simulink model "Control_Adap_1"  (R2021b)
settings: Solver=VariableStepAuto  StartTime=0.0  StopTime=50  RelTol=1e-3
settings Model: Creator=Alejandro  LastModifiedBy=cesar

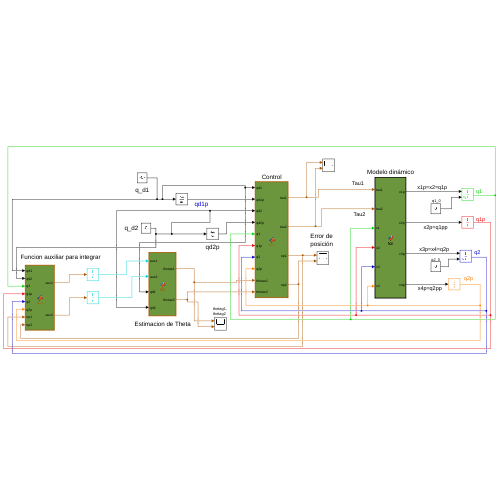
[thumbnail: Simulink's stored preview of the top-level diagram]
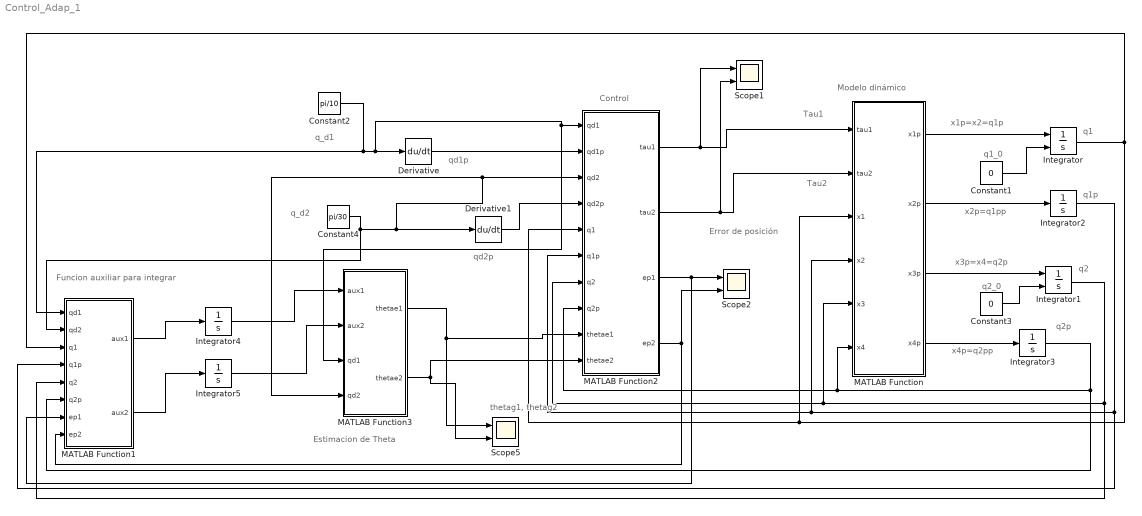
== system Control_Adap_1 ==
  note: Modelo dinámico
  note: q1_0
  note: q2p
  note: q2
  note: q1
  note: q_d2
  note: x3p=x4=q2p
  note: x2p=q1pp
  note: Tau2
  note: Error de posición
  note: x1p=x2=q1p
  note: x4p=q2pp
  note: Control
  note: qd1p
  note: Tau1
  note: q_d1
  note: qd2p
  note: q1p
  note: q2_0
  note: thetag1, thetag2
  note: Estimacion de Theta
  note: Funcion auxiliar para integrar
  Constant1 : Constant  Value=0
  Constant2 : Constant  Value=pi/10
  Constant3 : Constant  Value=0
  Constant4 : Constant  Value=pi/30
  Derivative : Derivative
  Derivative1 : Derivative
  Integrator : Integrator  InitialConditionSource=external
  Integrator1 : Integrator  InitialConditionSource=external
  Integrator{2..5} (4 alike) : Integrator
  MATLAB Function : MATLAB Function  TreatAsAtomicUnit=on
  MATLAB Function1 : MATLAB Function  TreatAsAtomicUnit=on
  MATLAB Function2 : MATLAB Function  TreatAsAtomicUnit=on
  MATLAB Function3 : MATLAB Function  TreatAsAtomicUnit=on
  Scope1 : Scope  NumInputPorts=2
  Scope2 : Scope  NumInputPorts=2
  Scope5 : Scope  NumInputPorts=2
  wires:
  Constant4/1 -> MATLAB Function1/2(qd2), Derivative1/1, MATLAB Function2/3(qd2), MATLAB Function3/4(qd2)
  Derivative/1 -> MATLAB Function2/2(qd1p)
  MATLAB Function3/1(thetae1) -> MATLAB Function2/9(thetae1), Scope5/1
  MATLAB Function2/1(tau1) -> Scope1/1, MATLAB Function/1(tau1)
  Constant2/1 -> MATLAB Function1/1(qd1), Derivative/1, MATLAB Function3/3(qd1), MATLAB Function2/1(qd1)
  MATLAB Function/4(x4p) -> Integrator3/1
  Constant3/1 -> Integrator1/2
  Integrator2/1 -> MATLAB Function1/4(q1p), MATLAB Function/4(x2), MATLAB Function2/6(q1p)
  MATLAB Function2/2(tau2) -> Scope1/2, MATLAB Function/2(tau2)
  Constant1/1 -> Integrator/2
  Integrator/1 -> MATLAB Function1/3(q1), MATLAB Function2/5(q1), MATLAB Function/3(x1)
  MATLAB Function/2(x2p) -> Integrator2/1
  MATLAB Function/3(x3p) -> Integrator1/1
  MATLAB Function/1(x1p) -> Integrator/1
  Integrator3/1 -> MATLAB Function1/6(q2p), MATLAB Function2/8(q2p), MATLAB Function/6(x4)
  Derivative1/1 -> MATLAB Function2/4(qd2p)
  Integrator1/1 -> MATLAB Function1/5(q2), MATLAB Function/5(x3), MATLAB Function2/7(q2)
  Integrator4/1 -> MATLAB Function3/1(aux1)
  MATLAB Function1/1(aux1) -> Integrator4/1
  MATLAB Function1/2(aux2) -> Integrator5/1
  Integrator5/1 -> MATLAB Function3/2(aux2)
  MATLAB Function3/2(thetae2) -> MATLAB Function2/10(thetae2), Scope5/2
  MATLAB Function2/3(ep1) -> MATLAB Function1/7(ep1), Scope2/1
  MATLAB Function2/4(ep2) -> Scope2/2, MATLAB Function1/8(ep2)

== matlab function Control_Adap_1/MATLAB Function1 ==
  data: qd1 input; qd2 input; q1 input; q1p input; q2 input; q2p input; aux1 output; aux2 output; ep1 input; ep2 input
function [aux1,aux2]= fcn(qd1,qd2,q1,q1p,q2,q2p,ep1,ep2)
% Parámetros
m1=6.5225;l1=0.26;lc1=0.0983;
g=9.81;I1=0.1213;
e0=5;
%---ERROR PARA EL ESLABÓN 1 ------
ep1=qd1-q1;     %qtilde
%ev1=qd1p-q1p;   %qtildepunto
%---ERROR PARA EL ESLABÓN 2 ------
ep2=qd2-q2;     %qtilde
%ev2=qd2p-q2p;   %qtildepunto
%------- VECTOR DE  ERROR DE POSICIÓN ------
ep=[ ep1;ep2];
%------- VECTOR DE  QP ------
qp=[ q1p;q2p];  
%---------- MATRIZ PHI_G -----------------------
phig=[l1*g*sin(qd1)   g*sin(qd1+qd2);
            0          g*sin(qd1+qd2)];    
a=l1*g*sin(qd1);
b=g*sin(qd1+qd2);
%------- Calcular de la variable auxiliar --------------
aux1=(e0/(1+norm(ep)))*(ep1-q1p);
aux2=(e0/(1+norm(ep)))*(ep2-q2p);

== matlab function Control_Adap_1/MATLAB Function ==
  data: tau1 input; x1p output; tau2 input; x1 input; x2 input; x3 input; x4 input; x2p output; x3p output; x4p output
function  [x1p,x2p,x3p,x4p] = fcn(tau1,tau2,x1,x2,x3,x4)
% Parámetros
m1=6.5225;I1=0.1213;
I2=0.0116;l1=0.26;
lc1=0.0983;lc2=0.0229;g=9.81;
qd1 = pi/10;
m2=2.0458;
l2 = 0.26;
%-------------------------------------------
M11=m1*lc1^2+m2*l1^2+m2*(l1^2+lc2^2+2*l1*lc2*cos(x3))+I1+I2;
M12=m2*lc2^2+m2*l1*lc2*cos(x3)+I2;
M21=m2*lc2^2+m2*l1*lc2*cos(x3)+I2;
M22=m2*lc2^2+I2;
C11=-m2*l1*lc2*sin(x3)*x4;
C12=-m2*l1*lc2*sin(x3)*(x2+x4);
C21=m2*l1*lc2*sin(x3)*x2;
C22=0;
g1=(m1*lc1+m2*l1)*g*sin(x1)+m2*lc2*g*sin(x1+x3); %+ m1*lc1*g*sin(qd1);
g2=m2*lc2*g*sin(x1+x3);
%------------------------
A=tau1-C11*x2-C12*x4-g1;
B=tau2-C21*x2-C22*x4-g2;
C=M11*M22-M12*M21;
%----------------------
%Modelo dinámico
x1p=x2;
x2p=(M22*A-M12*B)/C;
x3p=x4;
x4p=(-M21*A+M11*B)/C;

== matlab function Control_Adap_1/MATLAB Function2 ==
  data: qd1 input; qd1p input; qd2 input; qd2p input; q1 input; q1p input; q2 input; q2p input; thetae1 input; tau1 output; tau2 output; thetae2 input; ep1 output; ep2 output
function [tau1, tau2, ep1, ep2] = fcn(qd1,qd1p,qd2, ...
    qd2p,q1,q1p,q2,q2p,thetae1,thetae2)
% Parámetros 
m1=6.5225;l1=0.26;lc1=0.0983;
g=9.81;I1=0.1213;
%-------- MATRIZ DE Kp ------------  
Kp=[30 0;
    0 30];
%-------- MATRIZ DE Kv ---------------
Kv=[7 0;
    0 3];
%---ERROR PARA EL ESLABÓN 1 ------
ep1=qd1-q1;     %qtilde
ev1=qd1p-q1p;   %qtildepunto
%---ERROR PARA EL ESLABÓN 2 ------
ep2=qd2-q2;     %qtilde
ev2=qd2p-q2p;   %qtildepunto
%------- VECTOR DE  ERROR DE POSICIÓN ------
ep=[ ep1;
     ep2];
%------- VECTOR DE  ERROR DE velocidad ------
ev=[ ev1;
     ev2];
%------- VECTOR DE  QP ------
qp=[ q1p;
     q2p];  
%---------- MATRIZ PHI_G -----------------------
phig=[l1*g*sin(qd1)   g*sin(qd1+qd2);
            0         g*sin(qd1+qd2)];
% ---------------Matriz g_0(qd) ------------------
go=[m1*lc1*g*sin(qd1);
                   0];
%------- CALCULO DE TAU ------
tau1=30*ep1-7*q1p+l1*g*sin(qd1)*thetae1...
    +g*sin(qd1+qd2)*thetae2+m1*lc1*g*sin(qd1);
tau2=30*ep2-3*q2p+g*sin(qd1+qd2)*thetae2;

tau=[tau1;
     tau2];

== matlab function Control_Adap_1/MATLAB Function3 ==
  data: thetae1 output; aux1 input; aux2 input; qd1 input; qd2 input; thetae2 output
function [thetae1,thetae2]  = fcn(aux1,aux2, qd1, qd2)
%------- MATRIZ GAMMA ----------------
gamma=[500 0;
        0 10];
aux=[aux1;
     aux2];

m1=6.5225;l1=0.26;lc1=0.0983;
g=9.81;I1=0.1213;
e0=5;

%---------- Vector de theta_0 -----------------
thetae1=500*l1*g*sin(qd1)*aux1;
thetae2=10*g*sin(qd1+qd2)*aux1+10*g*sin(qd1+qd2)*aux2;
